simulink model "target_driver_2022_Ctrl_v_2_4_landing_2017a"  (R2017a)
settings: Solver=FixedStepDiscrete  StartTime=0.0  StopTime=13  FixedStep=0.0001  RelTol=1e-3  EnableMultiTasking=on
values from neighbouring files (symbols this model uses):
  a2_lb = -0.25    [target_driver_setup_2022_Ctrl_V_2_4.m]    (also in target_driver_setup_2022_Ctrl_V_2_4_christian.m)
  a2_openloop = -0    (= 0)    [target_driver_setup_2022_Ctrl_V_2_4.m]    (also in target_driver_setup_2022_Ctrl_V_2_4_christian.m)
  a2_ub = 0.25    [target_driver_setup_2022_Ctrl_V_2_4.m]    (also in target_driver_setup_2022_Ctrl_V_2_4_christian.m)
  adaptive_flag = 0    [target_driver_setup_2022_Ctrl_V_2_4.m]    (also in target_driver_setup_2022_Ctrl_V_2_4_christian.m)
  adaptive_gain = [gamma_adaptive, adaptive_roll_limit, adaptive_pitch_limit, adaptive_yaw_limit, c_2_adaptive, gamma_lateral_adaptive, adaptive_x_limit, adaptive_y_limit, adaptive_z_limit, c_1_adaptive]    [target_driver_setup_2022_Ctrl_V_2_4.m]    (also in target_driver_setup_2022_Ctrl_V_2_4_christian.m)
  adaptive_lateral_flag = 0    [target_driver_setup_2022_Ctrl_V_2_4.m]    (also in target_driver_setup_2022_Ctrl_V_2_4_christian.m)
  adaptive_pitch_init = 0    [target_driver_setup_2022_Ctrl_V_2_4.m]    (also in target_driver_setup_2022_Ctrl_V_2_4_christian.m)
  adaptive_pitch_limit = 0.1/(scale^2)    (= 1e-07)    [target_driver_setup_2022_Ctrl_V_2_4.m]    (also in target_driver_setup_2022_Ctrl_V_2_4_christian.m)
  adaptive_pitch_limit_low = -adaptive_pitch_limit    (= -1e-07)    [target_driver_setup_2022_Ctrl_V_2_4.m]    (also in target_driver_setup_2022_Ctrl_V_2_4_christian.m)
  adaptive_roll_init = 0    [target_driver_setup_2022_Ctrl_V_2_4.m]    (also in target_driver_setup_2022_Ctrl_V_2_4_christian.m)
  adaptive_roll_limit = 0.3/(scale^2)    (= 3e-07)    [target_driver_setup_2022_Ctrl_V_2_4.m]    (also in target_driver_setup_2022_Ctrl_V_2_4_christian.m)
  adaptive_roll_limit_low = -adaptive_roll_limit    (= -3e-07)    [target_driver_setup_2022_Ctrl_V_2_4.m]    (also in target_driver_setup_2022_Ctrl_V_2_4_christian.m)
  adaptive_x_init = 0    [target_driver_setup_2022_Ctrl_V_2_4.m]    (also in target_driver_setup_2022_Ctrl_V_2_4_christian.m)
  adaptive_x_limit = 0.15/(scale)    (= 0.00015)    [target_driver_setup_2022_Ctrl_V_2_4.m]    (also in target_driver_setup_2022_Ctrl_V_2_4_christian.m)
  adaptive_x_limit_low = -adaptive_x_limit    (= -0.00015)    [target_driver_setup_2022_Ctrl_V_2_4.m]    (also in target_driver_setup_2022_Ctrl_V_2_4_christian.m)
  adaptive_y_init = 0    [target_driver_setup_2022_Ctrl_V_2_4.m]    (also in target_driver_setup_2022_Ctrl_V_2_4_christian.m)
  adaptive_y_limit = 0.15/(scale)    (= 0.00015)    [target_driver_setup_2022_Ctrl_V_2_4.m]    (also in target_driver_setup_2022_Ctrl_V_2_4_christian.m)
  adaptive_y_limit_low = -adaptive_y_limit    (= -0.00015)    [target_driver_setup_2022_Ctrl_V_2_4.m]    (also in target_driver_setup_2022_Ctrl_V_2_4_christian.m)
  adaptive_yaw_init = 0    [target_driver_setup_2022_Ctrl_V_2_4.m]    (also in target_driver_setup_2022_Ctrl_V_2_4_christian.m)
  adaptive_yaw_limit = 0.035/(scale^2)    (= 3.5e-08)    [target_driver_setup_2022_Ctrl_V_2_4.m]    (also in target_driver_setup_2022_Ctrl_V_2_4_christian.m)
  adaptive_yaw_limit_low = -adaptive_yaw_limit    (= -3.5e-08)    [target_driver_setup_2022_Ctrl_V_2_4.m]    (also in target_driver_setup_2022_Ctrl_V_2_4_christian.m)
  adaptive_z_init = 0/scale    (= 0)    [target_driver_setup_2022_Ctrl_V_2_4.m]    (also in target_driver_setup_2022_Ctrl_V_2_4_christian.m)
  adaptive_z_limit = 0.20/(scale)    (= 0.0002)    [target_driver_setup_2022_Ctrl_V_2_4.m]    (also in target_driver_setup_2022_Ctrl_V_2_4_christian.m)
  adaptive_z_limit_low = -adaptive_z_limit/1    (= -0.0002)    [target_driver_setup_2022_Ctrl_V_2_4.m]    (also in target_driver_setup_2022_Ctrl_V_2_4_christian.m)
  att_s = 500    [target_driver_setup_2022_Ctrl_V_2_4.m]    (also in target_driver_setup_2022_Ctrl_V_2_4_christian.m)
  b_1_d_desired = [1,0,0]    [target_driver_setup_2022_Ctrl_V_2_4.m]    (also in target_driver_setup_2022_Ctrl_V_2_4_christian.m)
  closedloop_flag = 1    [target_driver_setup_2022_Ctrl_V_2_4.m]    (also in target_driver_setup_2022_Ctrl_V_2_4_christian.m)
  control_gain = [k_x,k_v, k_R, k_Omega, k_z, k_vz, k_Rx]    [target_driver_setup_2022_Ctrl_V_2_4.m]    (also in target_driver_setup_2022_Ctrl_V_2_4_christian.m)
  delay = delay-vicon_sample_cycle/2    [target_driver_setup_2022_Ctrl_V_2_4.m]    (also in target_driver_setup_2022_Ctrl_V_2_4_christian.m)
  drv_amp = 160    [target_driver_setup_2022_Ctrl_V_2_4.m]    (also in target_driver_setup_2022_Ctrl_V_2_4_christian.m)
  drv_bias = max_drv_bias    (= 300)    [target_driver_setup_2022_Ctrl_V_2_4.m]    (also in target_driver_setup_2022_Ctrl_V_2_4_christian.m)
  drv_pitch_left = 0    [target_driver_setup_2022_Ctrl_V_2_4.m]    (also in target_driver_setup_2022_Ctrl_V_2_4_christian.m)
  drv_pitch_right = 0    [target_driver_setup_2022_Ctrl_V_2_4.m]    (also in target_driver_setup_2022_Ctrl_V_2_4_christian.m)
  drv_roll = -2    [target_driver_setup_2022_Ctrl_V_2_4.m]    (also in target_driver_setup_2022_Ctrl_V_2_4_christian.m = 0)
  f_fin = f    (= 155)    [target_driver_setup_2022_Ctrl_V_2_4.m]    (also in target_driver_setup_2022_Ctrl_V_2_4_christian.m)
  f_int = f    (= 155)    [target_driver_setup_2022_Ctrl_V_2_4.m]    (also in target_driver_setup_2022_Ctrl_V_2_4_christian.m)
  g = 9.8    [target_driver_setup_2022_Ctrl_V_2_4.m]    (also in target_driver_setup_2022_Ctrl_V_2_4_christian.m)
  I_moment_vec = [Ixx, Iyy, Izz]    [target_driver_setup_2022_Ctrl_V_2_4.m]    (also in target_driver_setup_2022_Ctrl_V_2_4_christian.m)
  landing_flag = 0    [target_driver_setup_2022_Ctrl_V_2_4.m]    (also in target_driver_setup_2022_Ctrl_V_2_4_christian.m)
  landing_parameter = [start_delay+T,transition_rate, rising_time, falling_time, landing_rising_time, landing_z_decrease, landing_y_decrease, landing_x_decrease]    [target_driver_setup_2022_Ctrl_V_2_4.m]    (also in target_driver_setup_2022_Ctrl_V_2_4_christian.m = [start_delay+T, transition_rate, rising_time, falling_time, )
  low_bound = -8    [target_driver_setup_2022_Ctrl_V_2_4.m]    (also in target_driver_setup_2022_Ctrl_V_2_4_christian.m = -10)
  low_bound_eR = -0.8    [target_driver_setup_2022_Ctrl_V_2_4.m]    (also in target_driver_setup_2022_Ctrl_V_2_4_christian.m)
  low_bound_vx = -0.5    [target_driver_setup_2022_Ctrl_V_2_4.m]    (also in target_driver_setup_2022_Ctrl_V_2_4_christian.m)
  low_bound_vy = -0.5    [target_driver_setup_2022_Ctrl_V_2_4.m]    (also in target_driver_setup_2022_Ctrl_V_2_4_christian.m)
  low_bound_vz = -0.5    [target_driver_setup_2022_Ctrl_V_2_4.m]    (also in target_driver_setup_2022_Ctrl_V_2_4_christian.m)
  low_bound_x = -0.06    [target_driver_setup_2022_Ctrl_V_2_4.m]    (also in target_driver_setup_2022_Ctrl_V_2_4_christian.m)
  low_bound_y = -0.06    [target_driver_setup_2022_Ctrl_V_2_4.m]    (also in target_driver_setup_2022_Ctrl_V_2_4_christian.m)
  low_bound_z = -0.04    [target_driver_setup_2022_Ctrl_V_2_4.m]    (also in target_driver_setup_2022_Ctrl_V_2_4_christian.m)
  m = m+payload    (= 0.000124)    [target_driver_setup_2022_Ctrl_V_2_4.m]    (also in target_driver_setup_2022_Ctrl_V_2_4_christian.m = 0.000119)
  params_vec = [params_opt.delta_1, params_opt.delta_2, params_opt.delta_3, params_opt.gamma_1, params_opt.gamma_2, params_opt.gamma_3, params_opt.eta, params_opt.nu, params_opt.mu]'    [target_driver_setup_2022_Ctrl_V_2_4.m]    (also in target_driver_setup_2022_Ctrl_V_2_4_christian.m)
  phase = 0    [target_driver_setup_2022_Ctrl_V_2_4.m]    (also in target_driver_setup_2022_Ctrl_V_2_4_christian.m)
  r_desired = [default_x, default_y,z_desired]    [target_driver_setup_2022_Ctrl_V_2_4.m]    (also in target_driver_setup_2022_Ctrl_V_2_4_christian.m)
  roll_offset_angle = 0    [target_driver_setup_2022_Ctrl_V_2_4.m]    (also in target_driver_setup_2022_Ctrl_V_2_4_christian.m)
  running_time = start_delay+total_T    (= 8.5)    [target_driver_setup_2022_Ctrl_V_2_4.m]    (also in target_driver_setup_2022_Ctrl_V_2_4_christian.m = 8.4)
  running_time_control = start_delay_control+total_T+0.0    (= 8.6)    [target_driver_setup_2022_Ctrl_V_2_4.m]    (also in target_driver_setup_2022_Ctrl_V_2_4_christian.m = 8.5)
  start_delay = 2.0    (= 2)    [target_driver_setup_2022_Ctrl_V_2_4.m]    (also in target_driver_setup_2022_Ctrl_V_2_4_christian.m)
  start_delay_control = start_delay + ramp_delay    (= 2.1)    [target_driver_setup_2022_Ctrl_V_2_4.m]    (also in target_driver_setup_2022_Ctrl_V_2_4_christian.m)
  T = 0.5    [target_driver_setup_2022_Ctrl_V_2_4.m]    (also in target_driver_setup_2022_Ctrl_V_2_4_christian.m = 0.4)
  task_flag = 0    [target_driver_setup_2022_Ctrl_V_2_4.m]    (also in target_driver_setup_2022_Ctrl_V_2_4_christian.m)
  task_parameter = [radius_ref, frequency_ref, radius_ratio, lissajous_ratio, lissajous_delta, lissajous_amplitude_ratio,z_radius_ratio]    [target_driver_setup_2022_Ctrl_V_2_4.m]    (also in target_driver_setup_2022_Ctrl_V_2_4_christian.m)
  upp_bound = 8    [target_driver_setup_2022_Ctrl_V_2_4.m]    (also in target_driver_setup_2022_Ctrl_V_2_4_christian.m = 10)
  upp_bound_eR = 0.8    [target_driver_setup_2022_Ctrl_V_2_4.m]    (also in target_driver_setup_2022_Ctrl_V_2_4_christian.m)
  upp_bound_vx = 0.5    [target_driver_setup_2022_Ctrl_V_2_4.m]    (also in target_driver_setup_2022_Ctrl_V_2_4_christian.m)
  upp_bound_vy = 0.5    [target_driver_setup_2022_Ctrl_V_2_4.m]    (also in target_driver_setup_2022_Ctrl_V_2_4_christian.m)
  upp_bound_vz = 0.5    [target_driver_setup_2022_Ctrl_V_2_4.m]    (also in target_driver_setup_2022_Ctrl_V_2_4_christian.m)
  upp_bound_x = 0.06    [target_driver_setup_2022_Ctrl_V_2_4.m]    (also in target_driver_setup_2022_Ctrl_V_2_4_christian.m)
  upp_bound_y = 0.06    [target_driver_setup_2022_Ctrl_V_2_4.m]    (also in target_driver_setup_2022_Ctrl_V_2_4_christian.m)
  upp_bound_z = 0.04    [target_driver_setup_2022_Ctrl_V_2_4.m]    (also in target_driver_setup_2022_Ctrl_V_2_4_christian.m)
undefined symbols (not defined in the file or in its folder): A, Com1, DiscIntNeverNeededParam, left_mapping, left_mapping_F_to_Phi, lp_den, lp_num, none, right_mapping, right_mapping_F_to_Phi, vlp_den, vlp_num
libraries: simulink x25, xpcnilib x2, xpcseriallib x2, xpcutilitieslib x1
(part 2 of 4)

== system target_driver_2022_Ctrl_v_2_4_landing_2017a/Desired attitude and normalized error/Geometric derivative for Rd in SO(3) ==
  note: First order geometric derivative Rd in SO(3)
      | Patrick 2021 Mar
  Previous Averaged Rotation M : Inport
  Vicon Count : Inport  Port=2
  Current Averaged Rotation M : Inport  Port=3
  "Vicon Update Flag " : Inport  Port=4
  Demux1 : Demux  Outputs=3
  Demux2 : Demux  Outputs=3
  Discrete Derivative : simulink/Discrete/Discrete Derivative  gainval=1.0  ICPrevScaledInput=0.0  OutMin=[]  OutMax=[]  OutDataType=fixdt(1, 16)  OutScaling=2^-10  DoSatur=off
  "First order geometric derivative in SO(3) " : MATLAB Function  TreatAsAtomicUnit=on
  Mux1 : Mux  Inputs=3
  Mux2 : Mux  Inputs=3
  Previous Omega_d : Delay  DelayLength=1  InitialCondition=0
  filtered derivative1 : Subsystem
  filtered derivative5 : Subsystem
  Filtered Geometric derivative dRd in SO(3) : Outport
  Filtered Geometric derivative ddRd in SO(3)1 : Outport  Port=2
  wires:
  Previous Omega_d/1 -> "First order geometric derivative in SO(3) "/3(omega_d_prev)
  Previous Averaged Rotation M/1 -> "First order geometric derivative in SO(3) "/1(R_prev)
  Demux2/1 -> Mux2/1
  Demux2/2 -> Mux2/2
  filtered derivative5/1(Out1) -> Discrete Derivative/1, Demux2/1
  Mux2/1 -> Filtered Geometric derivative dRd in SO(3)/1
  "First order geometric derivative in SO(3) "/1(omega_d) -> Previous Omega_d/1, filtered derivative5/1(In1)
  Demux2/3 -> Mux2/3
  Current Averaged Rotation M/1 -> "First order geometric derivative in SO(3) "/2(R_cur)
  Vicon Count/1 -> "First order geometric derivative in SO(3) "/5(count)
  "Vicon Update Flag "/1 -> "First order geometric derivative in SO(3) "/4(update)
  Demux1/3 -> Mux1/3
  Mux1/1 -> Filtered Geometric derivative ddRd in SO(3)1/1
  Demux1/2 -> Mux1/2
  filtered derivative1/1(Out1) -> Demux1/1
  Demux1/1 -> Mux1/1
  Discrete Derivative/1 -> filtered derivative1/1(In1)

== system target_driver_2022_Ctrl_v_2_4_landing_2017a/Desired attitude and normalized error/saturated normalized error observation ==
  p : Inport
  v : Inport  Port=2
  R : Inport  Port=3
  omega : Inport  Port=4
  "omega_desired " : Inport  Port=5
  R_desired : Inport  Port=6
  r_desired : Inport  Port=7
  "v_desired " : Inport  Port=8
  "Saturated angular velocity eOmega " : Subsystem
  Saturated normalized eR : Subsystem
  "saturated normalized altitude error " : Subsystem
  "Normalized omega error " : Outport
  Normalized eR : Outport  Port=2
  "Normalized position error " : Outport  Port=3
  Normalized velocity error : Outport  Port=4
  wires:
  omega/1 -> "Saturated angular velocity eOmega "/1(omega)
  v/1 -> "saturated normalized altitude error "/1(averaged velocity)
  p/1 -> "saturated normalized altitude error "/2(averaged position)
  Saturated normalized eR/1(normalized eR) -> Normalized eR/1
  R/1 -> "Saturated angular velocity eOmega "/3(R_cur), Saturated normalized eR/1(Current averaged rotation M)
  R_desired/1 -> "Saturated angular velocity eOmega "/4(R_desired), Saturated normalized eR/2(R_desired)
  "Saturated angular velocity eOmega "/1(Normalized angular velocity) -> "Normalized omega error "/1
  "omega_desired "/1 -> "Saturated angular velocity eOmega "/2("omega_desired ")
  "saturated normalized altitude error "/1(Position error) -> "Normalized position error "/1
  "saturated normalized altitude error "/2(velocity_error) -> Normalized velocity error/1
  "v_desired "/1 -> "saturated normalized altitude error "/4(v_desired)
  r_desired/1 -> "saturated normalized altitude error "/3("r_desired ")

== system target_driver_2022_Ctrl_v_2_4_landing_2017a/Geometric Controller/Attitude Adaptive ==
  e_R : Inport
  e_Omega : Inport  Port=2
  Enable : Inport  Port=3
  Adaptive_flag : Inport  Port=4
  adaptive_gain : Inport  Port=5
  Adaptive Control : MATLAB Function  TreatAsAtomicUnit=on
  Compare To Zero : simulink/Logic and Bit Operations/Compare To Zero  relop=>  OutDataTypeStr=uint8  ZeroCross=off
  "Integrator " : DiscreteIntegrator  InitialConditionSource=external  InitialCondition=adaptive_roll_init  SampleTime=-1  LimitOutput=on  UpperSaturationLimit=adaptive_roll_limit  LowerSaturationLimit=adaptive_roll_limit_low  ICPrevOutput=DiscIntNeverNeededParam  ICPrevScaledInput=DiscIntNeverNeededParam
  Integrator 1 : DiscreteIntegrator  InitialConditionSource=external  InitialCondition=adaptive_pitch_init  SampleTime=-1  LimitOutput=on  UpperSaturationLimit=adaptive_pitch_limit  LowerSaturationLimit=adaptive_pitch_limit_low  ICPrevOutput=DiscIntNeverNeededParam  ICPrevScaledInput=DiscIntNeverNeededParam
  Integrator 2 : DiscreteIntegrator  InitialConditionSource=external  InitialCondition=adaptive_yaw_init  SampleTime=-1  LimitOutput=on  UpperSaturationLimit=adaptive_yaw_limit  LowerSaturationLimit=adaptive_yaw_limit_low  ICPrevOutput=DiscIntNeverNeededParam  ICPrevScaledInput=DiscIntNeverNeededParam
  Mux : Mux  Inputs=3
  Product{1,5..10} (7 alike) : Product  RndMeth=Zero
  adaptive_pitch_init : Constant  Value=adaptive_pitch_init
  "adaptive_roll_init " : Constant  Value=adaptive_roll_init
  adaptive_yaw_init : Constant  Value=adaptive_yaw_init
  adaptive_roll : Outport
  adaptive_pitch : Outport  Port=2
  adaptive_yaw : Outport  Port=3
  adaptive_attitude_control : Outport  Port=4
  wires:
  Product5/1 -> "Integrator "/1
  Adaptive Control/1(der_adaptive_torque_roll) -> Product5/2
  Product6/1 -> Integrator 1/1
  Adaptive Control/2(der_adaptive_torque_pitch) -> Product6/2
  Product7/1 -> Integrator 2/1
  Product8/1 -> adaptive_roll/1
  Adaptive Control/3(der_adaptive_torque_yaw) -> Product7/2
  Product9/1 -> adaptive_pitch/1
  Product10/1 -> adaptive_yaw/1
  Adaptive_flag/1 -> Compare To Zero/1
  Compare To Zero/1 -> Product1/1, Product10/1, Product9/1, Product8/1
  Integrator 2/1 -> Mux/3, Product10/2, Adaptive Control/3(current_adaptive_yaw)
  Integrator 1/1 -> Product9/2, Adaptive Control/2(current_adaptive_pitch), Mux/2
  "Integrator "/1 -> Product8/2, Adaptive Control/1(current_adaptive_roll), Mux/1
  adaptive_gain/1 -> Adaptive Control/6(adaptive_gain_limit)
  Mux/1 -> Product1/2
  "adaptive_roll_init "/1 -> "Integrator "/2
  adaptive_pitch_init/1 -> Integrator 1/2
  adaptive_yaw_init/1 -> Integrator 2/2
  e_R/1 -> Adaptive Control/4(e_R)
  Enable/1 -> Product7/1, Product6/1, Product5/1
  e_Omega/1 -> Adaptive Control/5(e_Omega)
  Product1/1 -> adaptive_attitude_control/1

== system target_driver_2022_Ctrl_v_2_4_landing_2017a/Geometric Controller/lateral adaptive ==
  e_x : Inport
  e_v : Inport  Port=2
  Enable : Inport  Port=3
  adaptive_gain : Inport  Port=4
  Adaptive_lateral_flag : Inport  Port=5
  Adaptive Control : MATLAB Function  TreatAsAtomicUnit=on
  Compare To Zero : simulink/Logic and Bit Operations/Compare To Zero  relop=>  OutDataTypeStr=uint8  ZeroCross=off
  "Integrator " : DiscreteIntegrator  InitialConditionSource=external  InitialCondition=adaptive_roll_init  SampleTime=-1  LimitOutput=on  UpperSaturationLimit=adaptive_x_limit  LowerSaturationLimit=adaptive_x_limit_low  ICPrevOutput=DiscIntNeverNeededParam  ICPrevScaledInput=DiscIntNeverNeededParam
  Integrator 1 : DiscreteIntegrator  InitialConditionSource=external  InitialCondition=adaptive_pitch_init  SampleTime=-1  LimitOutput=on  UpperSaturationLimit=adaptive_y_limit  LowerSaturationLimit=adaptive_y_limit_low  ICPrevOutput=DiscIntNeverNeededParam  ICPrevScaledInput=DiscIntNeverNeededParam
  Integrator 2 : DiscreteIntegrator  InitialConditionSource=external  InitialCondition=adaptive_yaw_init  SampleTime=-1  LimitOutput=on  UpperSaturationLimit=adaptive_z_limit  LowerSaturationLimit=adaptive_z_limit_low  ICPrevOutput=DiscIntNeverNeededParam  ICPrevScaledInput=DiscIntNeverNeededParam
  Mux : Mux  Inputs=3
  Product{1,5..10} (7 alike) : Product  RndMeth=Zero
  "adaptive_x_init " : Constant  Value=adaptive_x_init
  adaptive_y_init : Constant  Value=adaptive_y_init
  adaptive_z_init : Constant  Value=adaptive_z_init
  adaptive_lateral_control : Outport
  adaptive_x : Outport  Port=2
  adaptive_y : Outport  Port=3
  adaptive_z : Outport  Port=4
  wires:
  Product5/1 -> "Integrator "/1
  Adaptive Control/1(der_adaptive_torque_x) -> Product5/2
  Product6/1 -> Integrator 1/1
  Adaptive Control/2(der_adaptive_torque_y) -> Product6/2
  Product7/1 -> Integrator 2/1
  Adaptive Control/3(der_adaptive_torque_z) -> Product7/2
  adaptive_gain/1 -> Adaptive Control/6(adaptive_gain_limit)
  "adaptive_x_init "/1 -> "Integrator "/2
  adaptive_y_init/1 -> Integrator 1/2
  adaptive_z_init/1 -> Integrator 2/2
  e_x/1 -> Adaptive Control/4(e_x)
  Enable/1 -> Product7/1, Product6/1, Product5/1
  e_v/1 -> Adaptive Control/5(e_v)
  Compare To Zero/1 -> Product1/1, Product10/1, Product9/1, Product8/1
  Adaptive_lateral_flag/1 -> Compare To Zero/1
  "Integrator "/1 -> Adaptive Control/1(current_adaptive_x), Product8/2, Mux/1
  Integrator 1/1 -> Adaptive Control/2(current_adaptive_y), Product9/2, Mux/2
  Product9/1 -> adaptive_y/1
  Product8/1 -> adaptive_x/1
  Integrator 2/1 -> Product10/2, Mux/3, Adaptive Control/3(current_adaptive_z)
  Product10/1 -> adaptive_z/1
  Mux/1 -> Product1/2
  Product1/1 -> adaptive_lateral_control/1

== system target_driver_2022_Ctrl_v_2_4_landing_2017a/Observer for averaged system/Attitude Observer ==
  note: Attitude averaging and filtering using geometric average in Riemannian metric SO(3)
      |
      | Patrick 2021 Mar
  Vicon Update flag : Inport
  Raw Rotation : Inport  Port=2
  Vicon Count : Inport  Port=3
  Geometric Averaging Rotation Matix : Subsystem
  Geometric derivative in SO(3) : Subsystem
  "Averaged quaternion " : Outport
  Average Rotation Matrix : Outport  Port=2
  Raw quaternion : Outport  Port=3
  Geometric filtered derivative : Outport  Port=4
  wires:
  Vicon Count/1 -> Geometric derivative in SO(3)/2(Vicon Count)
  Raw Rotation/1 -> Geometric Averaging Rotation Matix/2(Current Rotation)
  Vicon Update flag/1 -> Geometric derivative in SO(3)/4("Vicon Update Flag "), Geometric Averaging Rotation Matix/1(Vicon Update flag)
  Geometric Averaging Rotation Matix/4(Previous Averaged Rotation Matrix) -> Geometric derivative in SO(3)/1(Previous Averaged Rotation M)
  Geometric derivative in SO(3)/1(Filtered Geometric derivative in SO(3)) -> Geometric filtered derivative/1
  Geometric Averaging Rotation Matix/3("Raw quaternion output ") -> Raw quaternion/1
  Geometric Averaging Rotation Matix/1(Averaged quaternion output) -> "Averaged quaternion "/1
  Geometric Averaging Rotation Matix/2("Averaged Rotation Matrix ") -> Average Rotation Matrix/1, Geometric derivative in SO(3)/3(Current Averaged Rotation M)

== system target_driver_2022_Ctrl_v_2_4_landing_2017a/Observer for averaged system/Euler derivative & filtered angular velocity  ==
  note: The skew symmetric structure is corrected from
      | the old angular velocity calculation.
      | Note from Patrick 2021 Mar
  "Rotation matrix " : Inport
  Angular velocity : MATLAB Function  TreatAsAtomicUnit=on
  Demux : Demux  Outputs=3
  Mux : Mux  Inputs=3
  filtered derivative : Subsystem
  Angular velocity_Euler : Outport
  Frob_norm error : Outport  Port=2
  wires:
  Demux/2 -> Mux/2
  Demux/3 -> Mux/3
  Mux/1 -> Angular velocity_Euler/1
  filtered derivative/1(Out1) -> Angular velocity/2(Rdot)
  Angular velocity/1(w) -> Demux/1
  Demux/1 -> Mux/1
  Angular velocity/2(Frob_error) -> Frob_norm error/1
  "Rotation matrix "/1 -> Angular velocity/1(R), filtered derivative/1(In1)

== system target_driver_2022_Ctrl_v_2_4_landing_2017a/Observer for averaged system/Position Observer ==
  "raw_position " : Inport
  vicon Update : Inport  Port=2
  Vicon Count : Inport  Port=3
  "Averaging position & velocity " : MATLAB Function  TreatAsAtomicUnit=on
  Delay10 : Delay  DelayLength=delay(2)  InitialCondition=0
  Delay11 : Delay  DelayLength=delay(3)  InitialCondition=0
  Delay14 : Delay  DelayLength=delay(4)  InitialCondition=0
  LowPassFiltere1 : Subsystem
  LowPassFiltere2 : Subsystem
  previous position : Delay  DelayLength=1  InitialCondition=0
  previous velocity : Delay  DelayLength=1  InitialCondition=0
  Average and filtered position : Outport
  Averaged and filtered velocity : Outport  Port=2
  wires:
  previous velocity/1 -> "Averaging position & velocity "/8(vout_prev)
  "Averaging position & velocity "/2(vout) -> previous velocity/1, LowPassFiltere2/1(In1)
  previous position/1 -> "Averaging position & velocity "/7(rout_prev)
  "raw_position "/1 -> "Averaging position & velocity "/4(r_cur), Delay14/1, Delay11/1, Delay10/1
  Delay14/1 -> "Averaging position & velocity "/3(r_prev3)
  Delay11/1 -> "Averaging position & velocity "/2(r_prev2)
  Delay10/1 -> "Averaging position & velocity "/1(r_prev)
  LowPassFiltere2/1(Out1) -> Averaged and filtered velocity/1
  "Averaging position & velocity "/1(rout) -> previous position/1, LowPassFiltere1/1(In1)
  LowPassFiltere1/1(Out1) -> Average and filtered position/1
  vicon Update/1 -> "Averaging position & velocity "/5(update)
  Vicon Count/1 -> "Averaging position & velocity "/6(count)

== system target_driver_2022_Ctrl_v_2_4_landing_2017a/Open_Closed_loop_selection/SIgnalForRamp_binary ==
  note: Should output 1 or -1,
      | so signal ramps UP to 1
      | or DOWN to 0.
  In1 : Inport
  Add : Sum  Inputs=+-
  Compare To Zero : simulink/Logic and Bit Operations/Compare To Zero  relop=>  OutDataTypeStr=uint8  ZeroCross=off
  Constant : Constant
  Data Type Conversion : DataTypeConversion  OutDataTypeStr=double
  Gain : Gain  Gain=2
  Out1 : Outport
  wires:
  In1/1 -> Compare To Zero/1
  Compare To Zero/1 -> Data Type Conversion/1
  Gain/1 -> Add/1
  Constant/1 -> Add/2
  Add/1 -> Out1/1
  Data Type Conversion/1 -> Gain/1

== system target_driver_2022_Ctrl_v_2_4_landing_2017a/Open_Closed_loop_selection/counter ==
  running time : Inport
  Add : Sum  Inputs=+-
  Compare To Zero : simulink/Logic and Bit Operations/Compare To Zero  relop=<  OutDataTypeStr=uint8  ZeroCross=off
  Product2 : Product  RndMeth=Zero
  SaturatingRamp : DiscreteIntegrator  gainval=1  SampleTime=-1  UpperSaturationLimit=1  LowerSaturationLimit=0  ICPrevOutput=DiscIntNeverNeededParam  ICPrevScaledInput=DiscIntNeverNeededParam
  constant : Constant
  start delay compare : simulink/Logic and Bit Operations/Compare To Constant  relop=>  const=start_delay  OutDataTypeStr=uint8
  enable : Outport
  wires:
  SaturatingRamp/1 -> Add/1, start delay compare/1
  running time/1 -> Add/2
  Add/1 -> Compare To Zero/1
  start delay compare/1 -> Product2/1
  Compare To Zero/1 -> Product2/2
  Product2/1 -> enable/1
  constant/1 -> SaturatingRamp/1

== system target_driver_2022_Ctrl_v_2_4_landing_2017a/Open_Closed_loop_selection/counter1 ==
  running time : Inport
  Add : Sum  Inputs=+-
  Compare To Zero : simulink/Logic and Bit Operations/Compare To Zero  relop=<  OutDataTypeStr=uint8  ZeroCross=off
  Product2 : Product  RndMeth=Zero
  SaturatingRamp : DiscreteIntegrator  gainval=1  SampleTime=-1  UpperSaturationLimit=1  LowerSaturationLimit=0  ICPrevOutput=DiscIntNeverNeededParam  ICPrevScaledInput=DiscIntNeverNeededParam
  constant : Constant
  start control delay compare : simulink/Logic and Bit Operations/Compare To Constant  relop=>  const=start_delay_control  OutDataTypeStr=uint8
  enable : Outport
  wires:
  SaturatingRamp/1 -> Add/1, start control delay compare/1
  running time/1 -> Add/2
  Add/1 -> Compare To Zero/1
  start control delay compare/1 -> Product2/1
  Compare To Zero/1 -> Product2/2
  Product2/1 -> enable/1
  constant/1 -> SaturatingRamp/1

== system target_driver_2022_Ctrl_v_2_4_landing_2017a/Open_Closed_loop_selection/timer1 ==
  SaturatingRamp : DiscreteIntegrator  gainval=1  SampleTime=-1  UpperSaturationLimit=1  LowerSaturationLimit=0  ICPrevOutput=DiscIntNeverNeededParam  ICPrevScaledInput=DiscIntNeverNeededParam
  constant : Constant
  time : Outport
  wires:
  SaturatingRamp/1 -> time/1
  constant/1 -> SaturatingRamp/1

== system target_driver_2022_Ctrl_v_2_4_landing_2017a/Phantom1/timer1 ==
  SaturatingRamp : DiscreteIntegrator  gainval=1  SampleTime=-1  UpperSaturationLimit=1  LowerSaturationLimit=0  ICPrevOutput=DiscIntNeverNeededParam  ICPrevScaledInput=DiscIntNeverNeededParam
  constant : Constant
  time : Outport
  wires:
  SaturatingRamp/1 -> time/1
  constant/1 -> SaturatingRamp/1

== system target_driver_2022_Ctrl_v_2_4_landing_2017a/Vicon Post Processing/Raw rotation matrix ==
  alpha : Inport
  beta : Inport  Port=2
  gamma : Inport  Port=3
  Mux : Mux  Inputs=9
  Rotation Matrix : Subsystem
  R : Outport
  wires:
  alpha/1 -> Rotation Matrix/1(alpha)
  beta/1 -> Rotation Matrix/2(beta)
  gamma/1 -> Rotation Matrix/3(gamma)
  Mux/1 -> R/1
  Rotation Matrix/1(R11) -> Mux/1
  Rotation Matrix/2(R12) -> Mux/2
  Rotation Matrix/3(R13) -> Mux/3
  Rotation Matrix/4(R21) -> Mux/4
  Rotation Matrix/5(R22) -> Mux/5
  Rotation Matrix/6(R23) -> Mux/6
  Rotation Matrix/7(R31) -> Mux/7
  Rotation Matrix/8(R32) -> Mux/8
  Rotation Matrix/9(R33) -> Mux/9

== system target_driver_2022_Ctrl_v_2_4_landing_2017a/Vicon Post Processing/Vicon Validity check ==
  "Rotation Matrix " : Inport
  Compare To Zero2 : simulink/Logic and Bit Operations/Compare To Zero  relop===  OutDataTypeStr=uint8
  Constant : Constant
  Data Type Conversion1 : DataTypeConversion  OutDataTypeStr=double
  Delay : Delay  DelayLength=1  InitialCondition=0
  Delay2 : Delay  DelayLength=1  InitialCondition=0
  MATLAB Function3 : MATLAB Function  TreatAsAtomicUnit=on
  SaturatingRamp : DiscreteIntegrator  gainval=sampling_f  ExternalReset=falling  SampleTime=-1  UpperSaturationLimit=1  LowerSaturationLimit=0  ICPrevOutput=DiscIntNeverNeededParam  ICPrevScaledInput=DiscIntNeverNeededParam
  type conv : DataTypeConversion  OutDataTypeStr=double
  "Vicon Update flag " : Outport
  Vicon Count : Outport  Port=2
  wires:
  Data Type Conversion1/1 -> Delay2/1, "Vicon Update flag "/1
  Delay/1 -> MATLAB Function3/1(R_prev)
  SaturatingRamp/1 -> Data Type Conversion1/1
  type conv/1 -> SaturatingRamp/2
  MATLAB Function3/1(y) -> Compare To Zero2/1
  Constant/1 -> SaturatingRamp/1
  Compare To Zero2/1 -> type conv/1
  "Rotation Matrix "/1 -> MATLAB Function3/2(R_cur), Delay/1
  Delay2/1 -> Vicon Count/1

== system target_driver_2022_Ctrl_v_2_4_landing_2017a/closed loop signal generator/Bias_Signal ==
  note: time constant = 0.002sec
  QuasiEnable : Inport
  BiasVolts : Inport  Port=2
  AveragedBias : Subsystem
  PreGain : Gain
  Product : Product  RndMeth=Zero
  SIgnalForRamp_binary : Subsystem
  SaturatingRamp : DiscreteIntegrator  gainval=10  SampleTime=-1  LimitOutput=on  UpperSaturationLimit=1  LowerSaturationLimit=0  ICPrevOutput=DiscIntNeverNeededParam  ICPrevScaledInput=DiscIntNeverNeededParam
  BiasD2A : Outport
  wires:
  PreGain/1 -> BiasD2A/1
  BiasVolts/1 -> AveragedBias/1(In1)
  QuasiEnable/1 -> SIgnalForRamp_binary/1(In1)
  SIgnalForRamp_binary/1(Out1) -> SaturatingRamp/1
  SaturatingRamp/1 -> Product/1
  AveragedBias/1(Out1) -> Product/2
  Product/1 -> PreGain/1

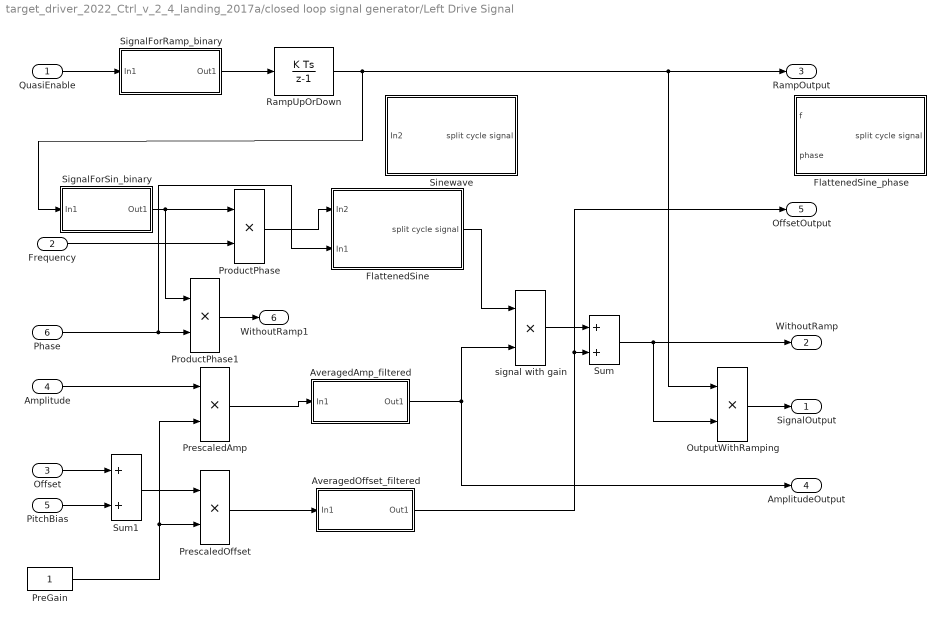
== system target_driver_2022_Ctrl_v_2_4_landing_2017a/closed loop signal generator/Left Drive Signal  ==
  QuasiEnable : Inport
  Frequency : Inport  Port=2
  Offset : Inport  Port=3
  Amplitude : Inport  Port=4
  PitchBias : Inport  Port=5
  Phase : Inport  Port=6
  AveragedAmp_filtered : Subsystem
  AveragedOffset_filtered : Subsystem
  FlattenedSine : Subsystem
  FlattenedSine_phase : Subsystem
  OutputWithRamping : Product  RndMeth=Zero
  PreGain : Constant
  PrescaledAmp : Product  RndMeth=Zero
  PrescaledOffset : Product  RndMeth=Zero
  ProductPhase : Product  RndMeth=Zero
  ProductPhase1 : Product  RndMeth=Zero
  RampUpOrDown : DiscreteIntegrator  gainval=10  SampleTime=-1  LimitOutput=on  UpperSaturationLimit=1  LowerSaturationLimit=0  ICPrevOutput=DiscIntNeverNeededParam  ICPrevScaledInput=DiscIntNeverNeededParam
  SignalForRamp_binary : Subsystem
  SignalForSin_binary : Subsystem
  Sinewave : Subsystem
  Sum : Sum
  Sum1 : Sum
  signal with gain : Product  RndMeth=Zero
  SignalOutput : Outport
  WithoutRamp : Outport  Port=2
  RampOutput : Outport  Port=3
  AmplitudeOutput : Outport  Port=4
  OffsetOutput : Outport  Port=5
  WithoutRamp1 : Outport  Port=6
  wires:
  PrescaledAmp/1 -> AveragedAmp_filtered/1(In1)
  Sum/1 -> OutputWithRamping/2, WithoutRamp/1
  RampUpOrDown/1 -> RampOutput/1, OutputWithRamping/1, SignalForSin_binary/1(In1)
  QuasiEnable/1 -> SignalForRamp_binary/1(In1)
  SignalForRamp_binary/1(Out1) -> RampUpOrDown/1
  Amplitude/1 -> PrescaledAmp/1
  signal with gain/1 -> Sum/1
  Frequency/1 -> ProductPhase/2
  SignalForSin_binary/1(Out1) -> ProductPhase/1, ProductPhase1/1
  AveragedOffset_filtered/1(Out1) -> Sum/2, OffsetOutput/1
  PrescaledOffset/1 -> AveragedOffset_filtered/1(In1)
  PreGain/1 -> PrescaledAmp/2, PrescaledOffset/2
  OutputWithRamping/1 -> SignalOutput/1
  AveragedAmp_filtered/1(Out1) -> signal with gain/2, AmplitudeOutput/1
  Sum1/1 -> PrescaledOffset/1
  Offset/1 -> Sum1/1
  PitchBias/1 -> Sum1/2
  Phase/1 -> ProductPhase1/2, FlattenedSine/2(In1)
  ProductPhase1/1 -> WithoutRamp1/1
  ProductPhase/1 -> FlattenedSine/1(In2)
  FlattenedSine/1(split cycle signal) -> signal with gain/1

== system target_driver_2022_Ctrl_v_2_4_landing_2017a/closed loop signal generator/Right Drive Signal ==
  QuasiEnable : Inport
  Frequency : Inport  Port=2
  Offset : Inport  Port=3
  Amplitude : Inport  Port=4
  PitchBias : Inport  Port=5
  AveragedAmp_filtered : Subsystem
  AveragedOffset_filtered : Subsystem
  FlattenedSine : Subsystem
  OutputWithRamping : Product  RndMeth=Zero
  PreGain : Constant
  PrescaledAmp : Product  RndMeth=Zero
  PrescaledOffset : Product  RndMeth=Zero
  ProductPhase : Product  RndMeth=Zero
  RampUpOrDown : DiscreteIntegrator  gainval=10  SampleTime=-1  LimitOutput=on  UpperSaturationLimit=1  LowerSaturationLimit=0  ICPrevOutput=DiscIntNeverNeededParam  ICPrevScaledInput=DiscIntNeverNeededParam
  SignalForRamp_binary : Subsystem
  SignalForSin_binary : Subsystem
  Sine Wave : Subsystem
  Sum : Sum
  Sum1 : Sum
  signal with gain : Product  RndMeth=Zero
  SignalOutput : Outport
  WithoutRamp : Outport  Port=2
  RampOutput : Outport  Port=3
  AmplitudeOutput : Outport  Port=4
  OffsetOutput : Outport  Port=5
  wires:
  PrescaledAmp/1 -> AveragedAmp_filtered/1(In1)
  Sum/1 -> OutputWithRamping/2, WithoutRamp/1
  RampUpOrDown/1 -> RampOutput/1, OutputWithRamping/1, SignalForSin_binary/1(In1)
  QuasiEnable/1 -> SignalForRamp_binary/1(In1)
  SignalForRamp_binary/1(Out1) -> RampUpOrDown/1
  signal with gain/1 -> Sum/1
  Frequency/1 -> ProductPhase/2
  SignalForSin_binary/1(Out1) -> ProductPhase/1
  AveragedOffset_filtered/1(Out1) -> Sum/2, OffsetOutput/1
  PrescaledOffset/1 -> AveragedOffset_filtered/1(In1)
  PreGain/1 -> PrescaledAmp/2, PrescaledOffset/2
  OutputWithRamping/1 -> SignalOutput/1
  AveragedAmp_filtered/1(Out1) -> signal with gain/2, AmplitudeOutput/1
  Sum1/1 -> PrescaledOffset/1
  Offset/1 -> Sum1/1
  PitchBias/1 -> Sum1/2
  Amplitude/1 -> PrescaledAmp/1
  FlattenedSine/1(split cycle signal) -> signal with gain/1
  ProductPhase/1 -> FlattenedSine/1(In2)

== system target_driver_2022_Ctrl_v_2_4_landing_2017a/closed loop signal generator/SignalSaturationLimit ==
  BiasMax : Inport
  SignalRaw : Inport  Port=2
  GainBias : Gain
  MaxOf : MinMax  Function=max  Inputs=2
  MinOf : MinMax  Inputs=2
  ground : Constant
  SignalSatd : Outport
  wires:
  BiasMax/1 -> GainBias/1
  SignalRaw/1 -> MinOf/2
  MinOf/1 -> MaxOf/1
  MaxOf/1 -> SignalSatd/1
  GainBias/1 -> MinOf/1
  ground/1 -> MaxOf/2

== system target_driver_2022_Ctrl_v_2_4_landing_2017a/closed loop signal generator/SignalSaturationLimit1 ==
  BiasMax : Inport
  SignalRaw : Inport  Port=2
  GainBias : Gain
  MaxOf : MinMax  Function=max  Inputs=2
  MinOf : MinMax  Inputs=2
  ground : Constant
  SignalSatd : Outport
  wires:
  BiasMax/1 -> GainBias/1
  SignalRaw/1 -> MinOf/2
  MinOf/1 -> MaxOf/1
  MaxOf/1 -> SignalSatd/1
  GainBias/1 -> MinOf/1
  ground/1 -> MaxOf/2

== system target_driver_2022_Ctrl_v_2_4_landing_2017a/signal generator a1/Bias_Signal ==
  note: time constant = 0.002sec
  QuasiEnable : Inport
  BiasVolts : Inport  Port=2
  AveragedBias : Subsystem
  PreGain : Gain
  Product : Product  RndMeth=Zero
  SIgnalForRamp_binary : Subsystem
  SaturatingRamp : DiscreteIntegrator  gainval=10  SampleTime=-1  LimitOutput=on  UpperSaturationLimit=1  LowerSaturationLimit=0  ICPrevOutput=DiscIntNeverNeededParam  ICPrevScaledInput=DiscIntNeverNeededParam
  BiasD2A : Outport
  wires:
  PreGain/1 -> BiasD2A/1
  BiasVolts/1 -> AveragedBias/1(In1)
  QuasiEnable/1 -> SIgnalForRamp_binary/1(In1)
  SIgnalForRamp_binary/1(Out1) -> SaturatingRamp/1
  SaturatingRamp/1 -> Product/1
  AveragedBias/1(Out1) -> Product/2
  Product/1 -> PreGain/1

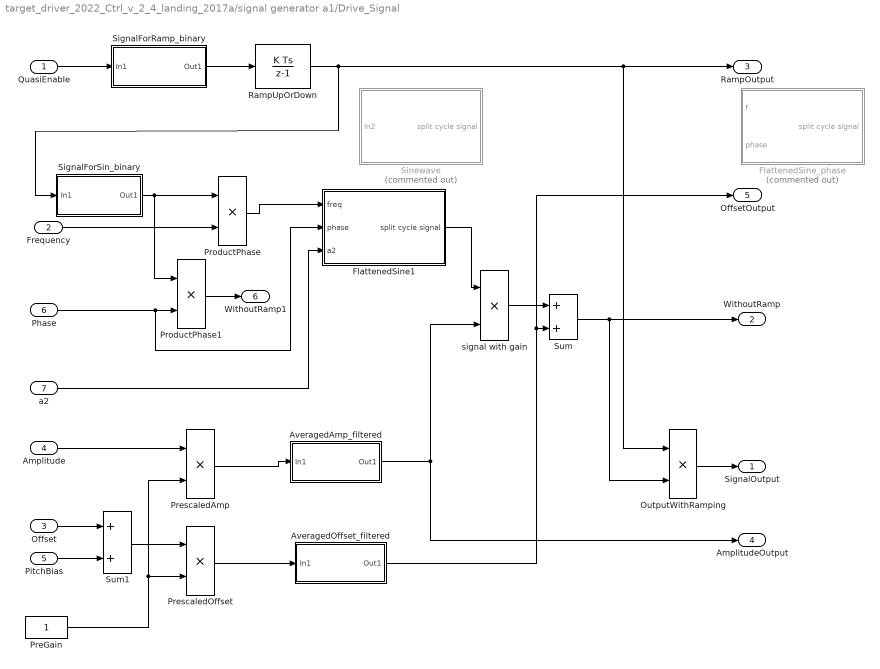
== system target_driver_2022_Ctrl_v_2_4_landing_2017a/signal generator a1/Drive_Signal ==
  QuasiEnable : Inport
  Frequency : Inport  Port=2
  Offset : Inport  Port=3
  Amplitude : Inport  Port=4
  PitchBias : Inport  Port=5
  Phase : Inport  Port=6
  "a2 " : Inport  Port=7
  AveragedAmp_filtered : Subsystem
  AveragedOffset_filtered : Subsystem
  FlattenedSine1 : Subsystem
  FlattenedSine_phase : Subsystem  Commented=on
  OutputWithRamping : Product  RndMeth=Zero
  PreGain : Constant
  PrescaledAmp : Product  RndMeth=Zero
  PrescaledOffset : Product  RndMeth=Zero
  ProductPhase : Product  RndMeth=Zero
  ProductPhase1 : Product  RndMeth=Zero
  RampUpOrDown : DiscreteIntegrator  gainval=10  SampleTime=-1  LimitOutput=on  UpperSaturationLimit=1  LowerSaturationLimit=0  ICPrevOutput=DiscIntNeverNeededParam  ICPrevScaledInput=DiscIntNeverNeededParam
  SignalForRamp_binary : Subsystem
  SignalForSin_binary : Subsystem
  Sinewave : Subsystem  Commented=on
  Sum : Sum
  Sum1 : Sum
  signal with gain : Product  RndMeth=Zero
  SignalOutput : Outport
  WithoutRamp : Outport  Port=2
  RampOutput : Outport  Port=3
  AmplitudeOutput : Outport  Port=4
  OffsetOutput : Outport  Port=5
  WithoutRamp1 : Outport  Port=6
  wires:
  PrescaledAmp/1 -> AveragedAmp_filtered/1(In1)
  Sum/1 -> OutputWithRamping/2, WithoutRamp/1
  RampUpOrDown/1 -> RampOutput/1, OutputWithRamping/1, SignalForSin_binary/1(In1)
  QuasiEnable/1 -> SignalForRamp_binary/1(In1)
  SignalForRamp_binary/1(Out1) -> RampUpOrDown/1
  Amplitude/1 -> PrescaledAmp/1
  signal with gain/1 -> Sum/1
  Frequency/1 -> ProductPhase/2
  SignalForSin_binary/1(Out1) -> ProductPhase/1, ProductPhase1/1
  AveragedOffset_filtered/1(Out1) -> Sum/2, OffsetOutput/1
  PrescaledOffset/1 -> AveragedOffset_filtered/1(In1)
  PreGain/1 -> PrescaledAmp/2, PrescaledOffset/2
  OutputWithRamping/1 -> SignalOutput/1
  AveragedAmp_filtered/1(Out1) -> signal with gain/2, AmplitudeOutput/1
  Sum1/1 -> PrescaledOffset/1
  Offset/1 -> Sum1/1
  PitchBias/1 -> Sum1/2
  Phase/1 -> FlattenedSine1/2(phase), ProductPhase1/2
  ProductPhase1/1 -> WithoutRamp1/1
  FlattenedSine1/1(split cycle signal) -> signal with gain/1
  ProductPhase/1 -> FlattenedSine1/1(freq)
  "a2 "/1 -> FlattenedSine1/3(a2)

== system target_driver_2022_Ctrl_v_2_4_landing_2017a/signal generator a1/Drive_Signal1 ==
  QuasiEnable : Inport
  Frequency : Inport  Port=2
  Offset : Inport  Port=3
  Amplitude : Inport  Port=4
  PitchBias : Inport  Port=5
  a2 : Inport  Port=6
  AveragedAmp_filtered : Subsystem
  AveragedOffset_filtered : Subsystem
  FlattenedSine1 : Subsystem
  OutputWithRamping : Product  RndMeth=Zero
  PreGain : Constant
  PrescaledAmp : Product  RndMeth=Zero
  PrescaledOffset : Product  RndMeth=Zero
  ProductPhase : Product  RndMeth=Zero
  RampUpOrDown : DiscreteIntegrator  gainval=10  SampleTime=-1  LimitOutput=on  UpperSaturationLimit=1  LowerSaturationLimit=0  ICPrevOutput=DiscIntNeverNeededParam  ICPrevScaledInput=DiscIntNeverNeededParam
  SignalForRamp_binary : Subsystem
  SignalForSin_binary : Subsystem
  Sine Wave : Subsystem  Commented=on
  Sum : Sum
  Sum1 : Sum
  signal with gain : Product  RndMeth=Zero
  SignalOutput : Outport
  WithoutRamp : Outport  Port=2
  RampOutput : Outport  Port=3
  AmplitudeOutput : Outport  Port=4
  OffsetOutput : Outport  Port=5
  wires:
  PrescaledAmp/1 -> AveragedAmp_filtered/1(In1)
  Sum/1 -> OutputWithRamping/2, WithoutRamp/1
  RampUpOrDown/1 -> RampOutput/1, OutputWithRamping/1, SignalForSin_binary/1(In1)
  QuasiEnable/1 -> SignalForRamp_binary/1(In1)
  SignalForRamp_binary/1(Out1) -> RampUpOrDown/1
  signal with gain/1 -> Sum/1
  Frequency/1 -> ProductPhase/2
  SignalForSin_binary/1(Out1) -> ProductPhase/1
  AveragedOffset_filtered/1(Out1) -> Sum/2, OffsetOutput/1
  PrescaledOffset/1 -> AveragedOffset_filtered/1(In1)
  PreGain/1 -> PrescaledAmp/2, PrescaledOffset/2
  OutputWithRamping/1 -> SignalOutput/1
  AveragedAmp_filtered/1(Out1) -> signal with gain/2, AmplitudeOutput/1
  Sum1/1 -> PrescaledOffset/1
  Offset/1 -> Sum1/1
  PitchBias/1 -> Sum1/2
  Amplitude/1 -> PrescaledAmp/1
  ProductPhase/1 -> FlattenedSine1/1(freq)
  FlattenedSine1/1(split cycle signal) -> signal with gain/1
  a2/1 -> FlattenedSine1/2(a2)

== system target_driver_2022_Ctrl_v_2_4_landing_2017a/signal generator a1/SignalSaturationLimit ==
  BiasMax : Inport
  SignalRaw : Inport  Port=2
  GainBias : Gain
  MaxOf : MinMax  Function=max  Inputs=2
  MinOf : MinMax  Inputs=2
  ground : Constant
  SignalSatd : Outport
  wires:
  BiasMax/1 -> GainBias/1
  SignalRaw/1 -> MinOf/2
  MinOf/1 -> MaxOf/1
  MaxOf/1 -> SignalSatd/1
  GainBias/1 -> MinOf/1
  ground/1 -> MaxOf/2

== system target_driver_2022_Ctrl_v_2_4_landing_2017a/signal generator a1/SignalSaturationLimit1 ==
  BiasMax : Inport
  SignalRaw : Inport  Port=2
  GainBias : Gain
  MaxOf : MinMax  Function=max  Inputs=2
  MinOf : MinMax  Inputs=2
  ground : Constant
  SignalSatd : Outport
  wires:
  BiasMax/1 -> GainBias/1
  SignalRaw/1 -> MinOf/2
  MinOf/1 -> MaxOf/1
  MaxOf/1 -> SignalSatd/1
  GainBias/1 -> MinOf/1
  ground/1 -> MaxOf/2

== system target_driver_2022_Ctrl_v_2_4_landing_2017a/signal generator a2/Bias_Signal ==
  note: time constant = 0.002sec
  QuasiEnable : Inport
  BiasVolts : Inport  Port=2
  AveragedBias : Subsystem
  PreGain : Gain
  Product : Product  RndMeth=Zero
  SIgnalForRamp_binary : Subsystem
  SaturatingRamp : DiscreteIntegrator  gainval=10  SampleTime=-1  LimitOutput=on  UpperSaturationLimit=1  LowerSaturationLimit=0  ICPrevOutput=DiscIntNeverNeededParam  ICPrevScaledInput=DiscIntNeverNeededParam
  BiasD2A : Outport
  wires:
  PreGain/1 -> BiasD2A/1
  BiasVolts/1 -> AveragedBias/1(In1)
  QuasiEnable/1 -> SIgnalForRamp_binary/1(In1)
  SIgnalForRamp_binary/1(Out1) -> SaturatingRamp/1
  SaturatingRamp/1 -> Product/1
  AveragedBias/1(Out1) -> Product/2
  Product/1 -> PreGain/1

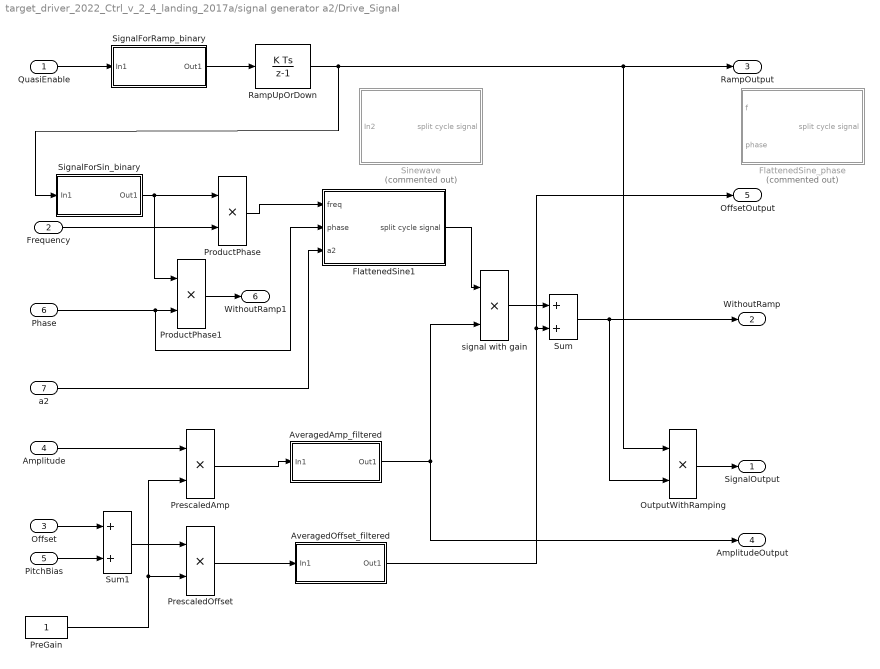
== system target_driver_2022_Ctrl_v_2_4_landing_2017a/signal generator a2/Drive_Signal ==
  QuasiEnable : Inport
  Frequency : Inport  Port=2
  Offset : Inport  Port=3
  Amplitude : Inport  Port=4
  PitchBias : Inport  Port=5
  Phase : Inport  Port=6
  "a2 " : Inport  Port=7
  AveragedAmp_filtered : Subsystem
  AveragedOffset_filtered : Subsystem
  FlattenedSine1 : Subsystem
  FlattenedSine_phase : Subsystem  Commented=on
  OutputWithRamping : Product  RndMeth=Zero
  PreGain : Constant
  PrescaledAmp : Product  RndMeth=Zero
  PrescaledOffset : Product  RndMeth=Zero
  ProductPhase : Product  RndMeth=Zero
  ProductPhase1 : Product  RndMeth=Zero
  RampUpOrDown : DiscreteIntegrator  gainval=10  SampleTime=-1  LimitOutput=on  UpperSaturationLimit=1  LowerSaturationLimit=0  ICPrevOutput=DiscIntNeverNeededParam  ICPrevScaledInput=DiscIntNeverNeededParam
  SignalForRamp_binary : Subsystem
  SignalForSin_binary : Subsystem
  Sinewave : Subsystem  Commented=on
  Sum : Sum
  Sum1 : Sum
  signal with gain : Product  RndMeth=Zero
  SignalOutput : Outport
  WithoutRamp : Outport  Port=2
  RampOutput : Outport  Port=3
  AmplitudeOutput : Outport  Port=4
  OffsetOutput : Outport  Port=5
  WithoutRamp1 : Outport  Port=6
  wires:
  PrescaledAmp/1 -> AveragedAmp_filtered/1(In1)
  Sum/1 -> OutputWithRamping/2, WithoutRamp/1
  RampUpOrDown/1 -> RampOutput/1, OutputWithRamping/1, SignalForSin_binary/1(In1)
  QuasiEnable/1 -> SignalForRamp_binary/1(In1)
  SignalForRamp_binary/1(Out1) -> RampUpOrDown/1
  Amplitude/1 -> PrescaledAmp/1
  signal with gain/1 -> Sum/1
  Frequency/1 -> ProductPhase/2
  SignalForSin_binary/1(Out1) -> ProductPhase/1, ProductPhase1/1
  AveragedOffset_filtered/1(Out1) -> Sum/2, OffsetOutput/1
  PrescaledOffset/1 -> AveragedOffset_filtered/1(In1)
  PreGain/1 -> PrescaledAmp/2, PrescaledOffset/2
  OutputWithRamping/1 -> SignalOutput/1
  AveragedAmp_filtered/1(Out1) -> signal with gain/2, AmplitudeOutput/1
  Sum1/1 -> PrescaledOffset/1
  Offset/1 -> Sum1/1
  PitchBias/1 -> Sum1/2
  Phase/1 -> FlattenedSine1/2(phase), ProductPhase1/2
  ProductPhase1/1 -> WithoutRamp1/1
  FlattenedSine1/1(split cycle signal) -> signal with gain/1
  ProductPhase/1 -> FlattenedSine1/1(freq)
  "a2 "/1 -> FlattenedSine1/3(a2)

== system target_driver_2022_Ctrl_v_2_4_landing_2017a/signal generator a2/Drive_Signal1 ==
  QuasiEnable : Inport
  Frequency : Inport  Port=2
  Offset : Inport  Port=3
  Amplitude : Inport  Port=4
  PitchBias : Inport  Port=5
  a2 : Inport  Port=6
  AveragedAmp_filtered : Subsystem
  AveragedOffset_filtered : Subsystem
  FlattenedSine1 : Subsystem
  OutputWithRamping : Product  RndMeth=Zero
  PreGain : Constant
  PrescaledAmp : Product  RndMeth=Zero
  PrescaledOffset : Product  RndMeth=Zero
  ProductPhase : Product  RndMeth=Zero
  RampUpOrDown : DiscreteIntegrator  gainval=10  SampleTime=-1  LimitOutput=on  UpperSaturationLimit=1  LowerSaturationLimit=0  ICPrevOutput=DiscIntNeverNeededParam  ICPrevScaledInput=DiscIntNeverNeededParam
  SignalForRamp_binary : Subsystem
  SignalForSin_binary : Subsystem
  Sine Wave : Subsystem  Commented=on
  Sum : Sum
  Sum1 : Sum
  signal with gain : Product  RndMeth=Zero
  SignalOutput : Outport
  WithoutRamp : Outport  Port=2
  RampOutput : Outport  Port=3
  AmplitudeOutput : Outport  Port=4
  OffsetOutput : Outport  Port=5
  wires:
  PrescaledAmp/1 -> AveragedAmp_filtered/1(In1)
  Sum/1 -> OutputWithRamping/2, WithoutRamp/1
  RampUpOrDown/1 -> RampOutput/1, OutputWithRamping/1, SignalForSin_binary/1(In1)
  QuasiEnable/1 -> SignalForRamp_binary/1(In1)
  SignalForRamp_binary/1(Out1) -> RampUpOrDown/1
  signal with gain/1 -> Sum/1
  Frequency/1 -> ProductPhase/2
  SignalForSin_binary/1(Out1) -> ProductPhase/1
  AveragedOffset_filtered/1(Out1) -> Sum/2, OffsetOutput/1
  PrescaledOffset/1 -> AveragedOffset_filtered/1(In1)
  PreGain/1 -> PrescaledAmp/2, PrescaledOffset/2
  OutputWithRamping/1 -> SignalOutput/1
  AveragedAmp_filtered/1(Out1) -> signal with gain/2, AmplitudeOutput/1
  Sum1/1 -> PrescaledOffset/1
  Offset/1 -> Sum1/1
  PitchBias/1 -> Sum1/2
  Amplitude/1 -> PrescaledAmp/1
  ProductPhase/1 -> FlattenedSine1/1(freq)
  FlattenedSine1/1(split cycle signal) -> signal with gain/1
  a2/1 -> FlattenedSine1/2(a2)

== system target_driver_2022_Ctrl_v_2_4_landing_2017a/signal generator a2/SignalSaturationLimit ==
  BiasMax : Inport
  SignalRaw : Inport  Port=2
  GainBias : Gain
  MaxOf : MinMax  Function=max  Inputs=2
  MinOf : MinMax  Inputs=2
  ground : Constant
  SignalSatd : Outport
  wires:
  BiasMax/1 -> GainBias/1
  SignalRaw/1 -> MinOf/2
  MinOf/1 -> MaxOf/1
  MaxOf/1 -> SignalSatd/1
  GainBias/1 -> MinOf/1
  ground/1 -> MaxOf/2

== system target_driver_2022_Ctrl_v_2_4_landing_2017a/signal generator a2/SignalSaturationLimit1 ==
  BiasMax : Inport
  SignalRaw : Inport  Port=2
  GainBias : Gain
  MaxOf : MinMax  Function=max  Inputs=2
  MinOf : MinMax  Inputs=2
  ground : Constant
  SignalSatd : Outport
  wires:
  BiasMax/1 -> GainBias/1
  SignalRaw/1 -> MinOf/2
  MinOf/1 -> MaxOf/1
  MaxOf/1 -> SignalSatd/1
  GainBias/1 -> MinOf/1
  ground/1 -> MaxOf/2

== system target_driver_2022_Ctrl_v_2_4_landing_2017a/Desired attitude and normalized error/Geometric derivative for Rd in SO(3)/filtered derivative1 ==
  In1 : Inport
  low pass3 : DiscreteTransferFcn  Numerator=vlp_num  Denominator=vlp_den
  Out1 : Outport
  wires:
  low pass3/1 -> Out1/1
  In1/1 -> low pass3/1

== system target_driver_2022_Ctrl_v_2_4_landing_2017a/Desired attitude and normalized error/Geometric derivative for Rd in SO(3)/filtered derivative5 ==
  In1 : Inport
  low pass3 : DiscreteTransferFcn  Numerator=lp_num  Denominator=lp_den
  Out1 : Outport
  wires:
  low pass3/1 -> Out1/1
  In1/1 -> low pass3/1

== system target_driver_2022_Ctrl_v_2_4_landing_2017a/Desired attitude and normalized error/saturated normalized error observation/Saturated angular velocity eOmega  ==
  omega : Inport
  "omega_desired " : Inport  Port=2
  R_cur : Inport  Port=3
  R_desired : Inport  Port=4
  Compute attitude error eR : MATLAB Function  TreatAsAtomicUnit=on
  Demux1 : Demux  Outputs=3
  Gain : Gain  Gain=2/(upp_bound-low_bound)
  Gain1 : Gain  Gain=2/(upp_bound-low_bound)
  Gain2 : Gain  Gain=2/(upp_bound-low_bound)
  Mux5 : Mux  Inputs=3
  Saturation1 : Saturate  UpperLimit=upp_bound  LowerLimit=low_bound
  Saturation2 : Saturate  UpperLimit=upp_bound  LowerLimit=low_bound
  Saturation3 : Saturate  UpperLimit=upp_bound  LowerLimit=low_bound
  Normalized angular velocity : Outport
  wires:
  Saturation1/1 -> Gain/1
  Mux5/1 -> Normalized angular velocity/1
  Saturation2/1 -> Gain1/1
  Gain/1 -> Mux5/1
  Gain1/1 -> Mux5/2
  "omega_desired "/1 -> Compute attitude error eR/4(omega_desired)
  Demux1/1 -> Saturation1/1
  R_desired/1 -> Compute attitude error eR/2(R_desired)
  R_cur/1 -> Compute attitude error eR/1(R_cur)
  omega/1 -> Compute attitude error eR/3(omega)
  Compute attitude error eR/1(y) -> Demux1/1
  Demux1/2 -> Saturation2/1
  Demux1/3 -> Saturation3/1
  Saturation3/1 -> Gain2/1
  Gain2/1 -> Mux5/3

== system target_driver_2022_Ctrl_v_2_4_landing_2017a/Desired attitude and normalized error/saturated normalized error observation/Saturated normalized eR ==
  Current averaged rotation M : Inport
  R_desired : Inport  Port=2
  Compute attitude error eR : MATLAB Function  TreatAsAtomicUnit=on
  Gain6 : Gain  Gain=2/(upp_bound_eR-low_bound_eR)
  Saturation4 : Saturate  UpperLimit=upp_bound_eR  LowerLimit=low_bound_eR
  normalized eR : Outport
  wires:
  Compute attitude error eR/1(y) -> Saturation4/1
  Saturation4/1 -> Gain6/1
  R_desired/1 -> Compute attitude error eR/2(R_desired)
  Gain6/1 -> normalized eR/1
  Current averaged rotation M/1 -> Compute attitude error eR/1(R_cur)
